simulink model "cassie_sim"  (R2016b)
settings: Solver=ode23  StartTime=simulationParameters.startTime  StopTime=15  FixedStep=0.0005  EnableMultiTasking=on
PreLoadFcn:
  | controller.util.simulationInitFcn;
InitFcn:
  | controller.util.simulationInitFcn;
StartFcn:
  | controller.util.simulationStartFcn;
StopFcn:
  | controller.util.simulationStopFcn;
undefined symbols (not defined in the file or in its folder): cassieEtherCatData, CassieParameters, ControlParams
libraries: SimulationLibrary x25, sm_lib x2, nesl_utility x1
settings Model: Creator=case  LastModifiedBy=gyk
settings SolverCC: ZeroCrossControl=DisableAll  InsertRTBMode=Always
settings DataIOCC: SaveOutput=off  SignalLogging=off  DSMLogging=off  SaveTime=off
settings OptimizationCC: DefaultParameterBehavior=Inlined  UseFloatMulNetSlope=on  InlineInvariantSignals=on  EfficientFloat2IntCast=on  LifeSpan=inf  SimCompilerOptimization=on  AccelVerboseBuild=on
settings DebuggingCC: ReadBeforeWriteMsg=DisableAll  WriteAfterWriteMsg=DisableAll  WriteAfterReadMsg=DisableAll  ParameterUnderflowMsg=error  ParameterTunabilityLossMsg=error  UniqueDataStoreMsg=error  AllowSymbolicDim=off  StrictBusMsg=ErrorOnBusTreatedAsVector  SFUnexpectedBacktrackingDiag=warning  SFNoUnconditionalDefaultTransitionDiag=warning  SFExecutionAtInitializationDiag=none
settings HardwareCC: TargetBitPerPointer=64  TargetBitPerSizeT=64  TargetBitPerPtrDiffT=64  TargetLongLongMode=on  TargetIntDivRoundTo=Zero  TargetEndianess=LittleEndian  TargetWordSize=64  TargetHWDeviceType=MATLAB Host  ProdEqTarget=off
settings ModelReferenceCC: UpdateModelReferenceTargets=IfOutOfDate  ModelReferenceNumInstancesAllowed=Zero  ModelReferenceMinAlgLoopOccurrences=on  PropagateSignalLabelsOutOfModel=off
settings RTWCC: BuildConfiguration=Faster Runs  CheckMdlBeforeBuild=Warning
settings CodeAppCC: GenerateComments=off  SimulinkBlockComments=off
settings GRTTargetCC: MatFileLogging=off  MultiInstanceERTCode=on  CodeInterfacePackaging=Reusable function  SupportNonFinite=off  GenerateAllocFcn=on
settings ConfigComp: CovMetricSettings=dw  CovHtmlReporting=on  CovSaveCumulativeToWorkspaceVar=on  CovSaveSingleToWorkspaceVar=on  CovExternalEMLEnable=off
settings ExplorerConfigSet: InternalSimMechanicsExplorerSettings="<ExplorerConfiguration><canonicalview>default</canonicalview><AnimationSetting><BasePlaybackSpeed>1.0</BasePlaybackSpeed><PlaybackSpeedFactor>1.0</PlaybackSpeedFactor></AnimationSetting><TilePanel><TileInfo><Tiles Columns=\"1\" Count=\"1\" Rows=\"1\"><Column Left=\"2\" Weight=\"1\"/><Column Left=\"1053\"/><Row Top=\"2\" Weight=\"1\"/><Row Top=\"486\"/><Tile Height=\"1\" Width=\"1\" X=\"0\" Y=\"0\"/></Tiles></TileInfo><SceneInfo><SceneViewer><BGColor><R>0.60000002384185791</R><G>0.60000002384185791</G><B>0.60000002384185791</B></BGColor><Camera><DoPerspective>on</DoPerspective><Position><X>1.5163613923952763</X><Y>-1.4988060678602755</Y><Z>0.66118837525886986</Z></Position><Center><X>0.016361392395276342</X><Y>0.0011939321397245184</Y><Z>0.16118837525886986</Z></Center><Up><X>0</X><Y>0</Y><Z>1</Z></Up><ViewLimDist>1</ViewLimDist><YLim>0.46630765815499858</YLim><XLim>1.0229317469421231</XLim></Camera></SceneViewer></SceneInfo></TilePanel><MechEditorPanel><Cameras><Camera><Id>Camera1</Id><Value><Name>Tracking Camera</Name><NativeCamera><PositionTrackingFeature>Cassie_V2_Simulation_Subsystem.Cassie_Multibody_Subsystem.Pelvis.Tracking_Camera.F</PositionTrackingFeature><CenterTrackingFeature>Cassie_V2_Simulation_Subsystem.Cassie_Multibody_Subsystem.Pelvis.Tracking_Camera_Target.F</CenterTrackingFeature><UpVectorTrackingFeature>Cassie_V2_Simulation_Subsystem.Cassie_Multibody_Subsystem.Pelvis.Tracking_Camera_Target.F</UpVectorTrackingFeature><CenterTrackingOrigin>on</CenterTrackingOrigin><UpVectorTrackingDirection>+Z</UpVectorTrackingDirection></NativeCamera></Value></Camera><Camera><Id>Camera2</Id><Value><Name>Fixed Camera</Name><NativeCamera><PositionTrackingFeature>Cassie_V2_Simulation_Subsystem.Cassie_Multibody_Subsystem.Pelvis.Fixed_Camera.F</PositionTrackingFeature><CenterTrackingFeature>Cassie_V2_Simulation_Subsystem.Cassie_Multibody_Subsystem.Pelvis.Fixed_Camera_Target.F</CenterTrackingFeature><UpVectorTrackingFeature>Cassie_V2_Simulation_Subsystem.Cassie_Multibody_Subsystem.Pelvis.Fixed_Camera_Target.F</UpVectorTrackingFeature><CenterTrackingOrigin>on</CenterTrackingOrigin><UpVectorTrackingDirection>+Z</UpVectorTrackingDirection></NativeCamera></Value></Camera></Cameras><GfxPanelCameraMap><MapElement CameraMLId=\"Camera1\" GfxPanelIndex=\"0\"/></GfxPanelCameraMap><VideoCreator><PlaybackSpeedRatio>1.0</PlaybackSpeedRatio><FrameRate>30</FrameRate><VideoFormat>Motion JPEG AVI</VideoFormat><FrameSize>auto</FrameSize></VideoCreator></MechEditorPanel></ExplorerConfiguration>"

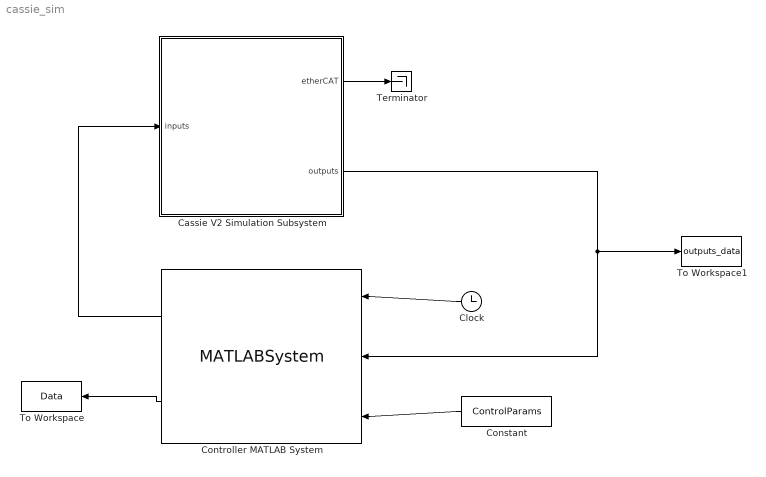
== system cassie_sim ==
  Cassie V2 Simulation Subsystem : Subsystem  VariantControl=(default)
      mask Display: image('CassieV2.png');
  Clock : Clock
  Constant : Constant  Value=ControlParams  OutDataTypeStr=Bus: cassieControlParamsBus
  Controller MATLAB System : MATLABSystem  System=controller.Controller  SimulateUsing=Interpreted execution
      mask Type: controller.Controller
      mask Display:
      | disp('Controller');
      | port_label('input',1,'t');
      | port_label('input',2,'outputs');
      | port_label('input',3,'ControlParams');
      | port_label('output',1,'inputs');
      | port_label('output',2,'Data');
  Terminator : Terminator
  To Workspace : ToWorkspace  VariableName=Data  SaveFormat=Timeseries  SampleTime=-1
  To Workspace1 : ToWorkspace  VariableName=outputs_data  SaveFormat=Timeseries  SampleTime=-1
  wires:
  Controller MATLAB System/1 -> Cassie V2 Simulation Subsystem/1(inputs)
  Cassie V2 Simulation Subsystem/1(etherCAT) -> Terminator/1
  Constant/1 -> Controller MATLAB System/3
  Clock/1 -> Controller MATLAB System/1
  Controller MATLAB System/2 -> To Workspace/1
  Cassie V2 Simulation Subsystem/2(outputs) -> To Workspace1/1, Controller MATLAB System/2

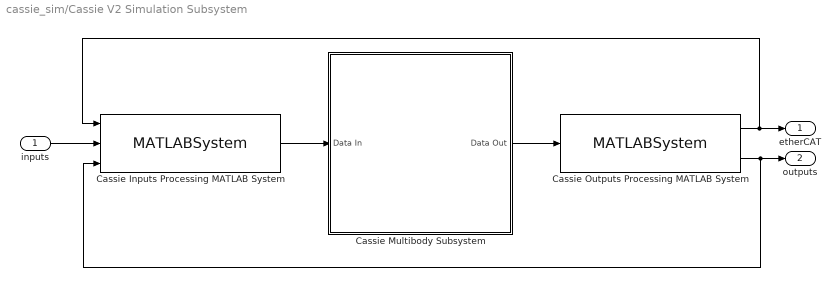
== system cassie_sim/Cassie V2 Simulation Subsystem ==
  inputs : Inport  OutDataTypeStr=Bus: cassieInputsBus  SampleTime=CassieParameters.etherCatSampleTime
  Cassie Inputs Processing MATLAB System : MATLABSystem  System=ProcessInputsSimulation  SimulateUsing=Code generation
      mask Type: ProcessInputsSimulation
      mask Display:
      | disp('ProcessInputsSimulation');
      | port_label('input',1,'etherCat');
      | port_label('input',2,'inputs');
      | port_label('input',3,'outputs');
      | port_label('output',1,'etherCat');
  Cassie Multibody Subsystem : Subsystem
      mask Display: image('CassieV2.png');
  Cassie Outputs Processing MATLAB System : MATLABSystem  System=ProcessOutputsSimulation  SimulateUsing=Code generation
      mask Type: ProcessOutputsSimulation
      mask Display:
      | disp('ProcessOutputsSimulation');
      | port_label('input',1,'etherCat');
      | port_label('output',1,'etherCat');
      | port_label('output',2,'outputs');
  etherCAT : Outport  OutDataTypeStr=Bus: cassieEtherCatBus  SampleTime=CassieParameters.etherCatSampleTime
  outputs : Outport  Port=2  OutDataTypeStr=Bus: cassieOutputsBus  SampleTime=CassieParameters.etherCatSampleTime
  wires:
  Cassie Multibody Subsystem/1(Data Out) -> Cassie Outputs Processing MATLAB System/1
  Cassie Outputs Processing MATLAB System/2 -> outputs/1, Cassie Inputs Processing MATLAB System/3
  Cassie Outputs Processing MATLAB System/1 -> etherCAT/1, Cassie Inputs Processing MATLAB System/1
  Cassie Inputs Processing MATLAB System/1 -> Cassie Multibody Subsystem/1(Data In)
  inputs/1 -> Cassie Inputs Processing MATLAB System/2

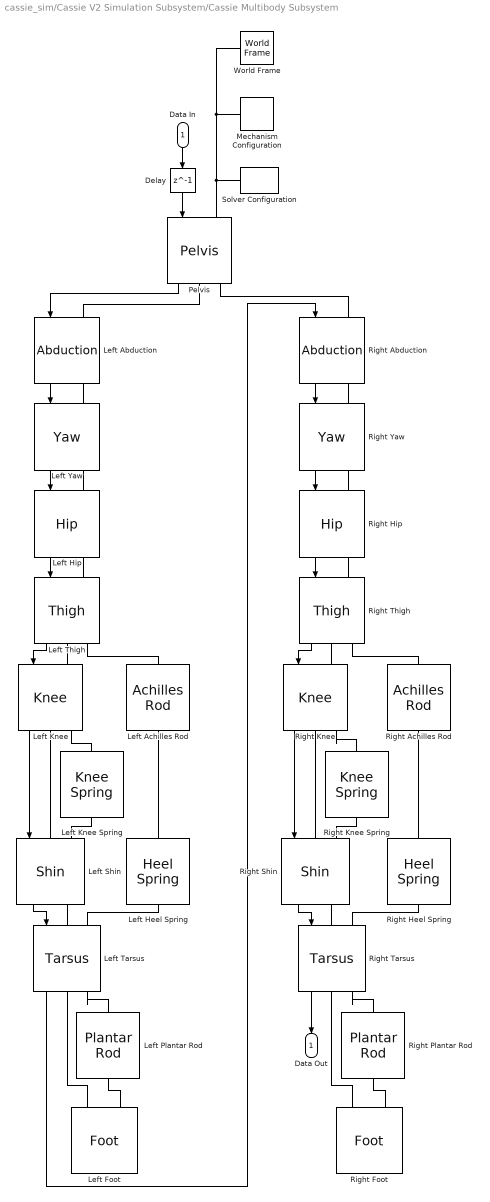
== system cassie_sim/Cassie V2 Simulation Subsystem/Cassie Multibody Subsystem ==
  Data In : Inport  PortDimensions=1
  Delay : Delay  DelayLength=1  InitialCondition=cassieEtherCatData  InputProcessing=Inherited  SampleTime=CassieParameters.etherCatSampleTime
  Left Abduction : SimulationLibrary/Abduction  side=Left
  Left Achilles Rod : SimulationLibrary/Achilles Rod  SystemSampleTime=-1
  Left Foot : SimulationLibrary/Foot  side=Left
  Left Heel Spring : SimulationLibrary/Heel Spring
  Left Hip : SimulationLibrary/Hip  side=Left
  Left Knee : SimulationLibrary/Knee  side=Left
  Left Knee Spring : SimulationLibrary/Knee Spring
  Left Plantar Rod : SimulationLibrary/Plantar Rod  SystemSampleTime=-1
  Left Shin : SimulationLibrary/Shin  side=Left
  Left Tarsus : SimulationLibrary/Tarsus  side=Left
  Left Thigh : SimulationLibrary/Thigh  side=Left
  Left Yaw : SimulationLibrary/Yaw  side=Left
  Mechanism Configuration : sm_lib/Utilities/Mechanism Configuration  UniformGravity=Constant  GravityVector=simulationParameters.gravity  GravityUnits=m/s^2  LinearizationDelta=0.001
  Pelvis : SimulationLibrary/Pelvis  SystemSampleTime=-1
  Right Abduction : SimulationLibrary/Abduction  side=Right
  Right Achilles Rod : SimulationLibrary/Achilles Rod  SystemSampleTime=-1
  Right Foot : SimulationLibrary/Foot  side=Right
  Right Heel Spring : SimulationLibrary/Heel Spring
  Right Hip : SimulationLibrary/Hip  side=Right
  Right Knee : SimulationLibrary/Knee  side=Right
  Right Knee Spring : SimulationLibrary/Knee Spring
  Right Plantar Rod : SimulationLibrary/Plantar Rod  SystemSampleTime=-1
  Right Shin : SimulationLibrary/Shin  side=Right
  Right Tarsus : SimulationLibrary/Tarsus  side=Right
  Right Thigh : SimulationLibrary/Thigh  side=Right
  Right Yaw : SimulationLibrary/Yaw  side=Right
  Solver Configuration : nesl_utility/Solver Configuration  PhysicalDomain=network_engine_domain  SubClassName=solver  LeftPortType=input  RightPortType=generic  Accelerate=off  Tones=[]  Harmonics=[]  SimulateNoise=off  Profile=off  UseLocalSampling=off  EnableSwitchedLinearOptims=on  FrequencyDomain=off  UseCCode=off  RelTol=0.001  AbsTol=1e-06  MinStep=1e-09  ToWorkspace=off  RevertToSquareIcSolve=off  NumHomotopyIterations=100  PhasorMode=off  PhasorModeNumHarmonics=1  OverrideAbsTol=off  DoDC=off  ResidualTolerance=1e-09  UseLocalSolver=off  LocalSolverChoice=NE_BACKWARD_EULER_ADVANCER  LocalSolverSampleTime=0.001  DoFixedCost=off  MaxNonlinIter=3  MaxModeIter=2  LinearAlgebra=Sparse  DelaysMemoryBudget=1024  AutomaticFiltering=on  FilteringTimeConstant=0.001
  World Frame : sm_lib/Frames and Transforms/World Frame
  Data Out : Outport  PortDimensions=1
  wires:
  Right Tarsus/1 -> Data Out/1
  Right Shin/1 -> Right Tarsus/1
  Left Tarsus/1 -> Right Abduction/1
  Left Shin/1 -> Left Tarsus/1
  Right Knee/1 -> Right Shin/1
  Pelvis/1 -> Left Abduction/1
  Delay/1 -> Pelvis/1
  Left Knee/1 -> Left Shin/1
  Right Thigh/1 -> Right Knee/1
  Left Thigh/1 -> Left Knee/1
  Right Hip/1 -> Right Thigh/1
  Right Yaw/1 -> Right Hip/1
  Left Hip/1 -> Left Thigh/1
  Left Yaw/1 -> Left Hip/1
  Left Abduction/1 -> Left Yaw/1
  Right Abduction/1 -> Right Yaw/1
  Data In/1 -> Delay/1
  connections:
  Right Foot/LConn2 -- Right Plantar Rod/RConn1
  Left Foot/LConn2 -- Left Plantar Rod/RConn1
  Right Tarsus/LConn2 -- Right Heel Spring/LConn1
  Right Tarsus/LConn1 -- Right Shin/RConn1
  Right Tarsus/RConn1 -- Right Foot/LConn1
  Right Tarsus/RConn2 -- Right Plantar Rod/LConn1
  Left Abduction/LConn1 -- Pelvis/RConn1
  Right Abduction/LConn1 -- Pelvis/RConn2
  Left Tarsus/RConn1 -- Left Foot/LConn1
  Left Tarsus/RConn2 -- Left Plantar Rod/LConn1
  Left Tarsus/LConn2 -- Left Heel Spring/LConn1
  Left Tarsus/LConn1 -- Left Shin/RConn1
  Right Heel Spring/RConn1 -- Right Achilles Rod/RConn1
  Right Shin/LConn1 -- Right Knee/RConn1
  Right Shin/LConn2 -- Right Knee Spring/RConn1
  Right Knee/RConn2 -- Right Knee Spring/LConn1
  Left Achilles Rod/RConn1 -- Left Heel Spring/RConn1
  Left Shin/LConn1 -- Left Knee/RConn1
  Left Shin/LConn2 -- Left Knee Spring/RConn1
  Left Knee/RConn2 -- Left Knee Spring/LConn1
  Right Thigh/RConn2 -- Right Achilles Rod/LConn1
  Right Knee/LConn1 -- Right Thigh/RConn1
  Left Thigh/RConn2 -- Left Achilles Rod/LConn1
  Left Knee/LConn1 -- Left Thigh/RConn1
  Right Thigh/LConn1 -- Right Hip/RConn1
  Right Hip/LConn1 -- Right Yaw/RConn1
  Left Thigh/LConn1 -- Left Hip/RConn1
  Left Hip/LConn1 -- Left Yaw/RConn1
  Right Yaw/LConn1 -- Right Abduction/RConn1
  Left Yaw/LConn1 -- Left Abduction/RConn1
  World Frame/RConn1 -- Mechanism Configuration/RConn1 -- Pelvis/LConn1 -- Solver Configuration/RConn1
